simulink model "compensacion_digital"  (R2014b)
settings: Solver=ode45  StartTime=0.0  StopTime=4  RelTol=1e-3
settings Model: Creator=Javi  LastModifiedBy=Javi

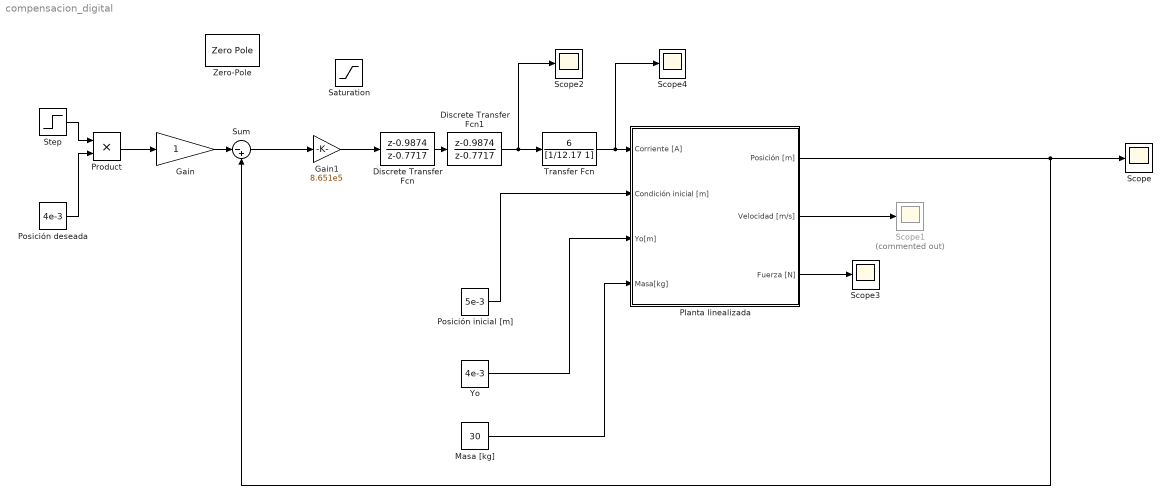
== system compensacion_digital ==
  Discrete Transfer Fcn : DiscreteTransferFcn  Numerator=[1 -0.9874]  Denominator=[1 -0.7717]  SampleTime=1/3.5e3
  Discrete Transfer Fcn1 : DiscreteTransferFcn  Numerator=[1 -0.9874]  Denominator=[1 -0.7717]
  Gain : Gain
  Gain1 : Gain  Gain=8.651e5
  "Masa [kg] " : Constant  Value=30
  Planta linealizada : Subsystem
  Posición deseada : Constant  Value=4e-3
  "Posición inicial [m] " : Constant  Value=5e-3
  Product : Product
  Saturation : Saturate  UpperLimit=5  LowerLimit=-inf
  Scope{,2..4} (4 alike) : Scope
      Scope settings: TimeRange=4  YMin=0  YMax=0.014
      Scope2 settings: TimeRange=0.005185185185185187  YMin=-3500000  YMax=500000  SaveName=ScopeData2
      Scope3 settings: TimeRange=4  YMin=-400000  YMax=600000  SaveName=ScopeData3
      Scope4 settings: TimeRange=0.005185185185185187  YMin=-3500000  YMax=500000  SaveName=ScopeData4
  Scope1 : Scope  Commented=on
  Step : Step  Time=0.01  SampleTime=0
  Sum : Sum  Inputs=|-+
  Transfer Fcn : TransferFcn  Numerator=[6]  Denominator=[1/12.17 1]
  "Yo " : Constant  Value=4e-3
  Zero-Pole : ZeroPole  Zeros=[-221.7 -221.7]  Poles=[-4511 -4511]  Gain=8.28e5
  wires:
  "Posición inicial [m] "/1 -> Planta linealizada/2("Condición inicial [m] ")
  "Yo "/1 -> Planta linealizada/3(Yo[m])
  "Masa [kg] "/1 -> Planta linealizada/4("Masa[kg] ")
  Planta linealizada/2(Velocidad [m/s]) -> Scope1/1
  Gain/1 -> Sum/1
  Planta linealizada/1(Posición [m]) -> Sum/2, Scope/1
  Transfer Fcn/1 -> Scope4/1, Planta linealizada/1(Corriente [A])
  Planta linealizada/3(Fuerza [N]) -> Scope3/1
  Discrete Transfer Fcn1/1 -> Scope2/1, Transfer Fcn/1
  Step/1 -> Product/1
  Posición deseada/1 -> Product/2
  Product/1 -> Gain/1
  Gain1/1 -> Discrete Transfer Fcn/1
  Sum/1 -> Gain1/1
  Discrete Transfer Fcn/1 -> Discrete Transfer Fcn1/1

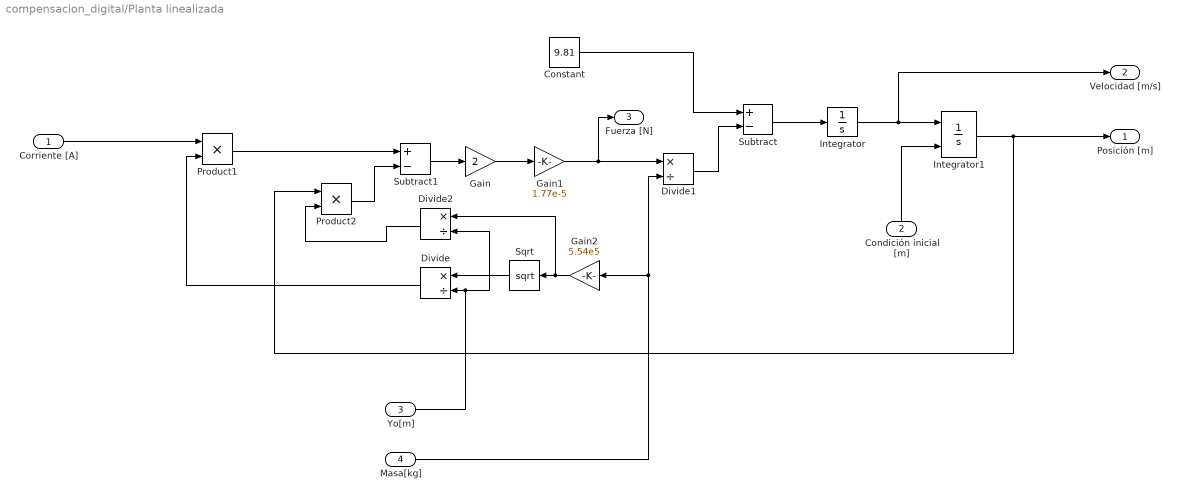
== system compensacion_digital/Planta linealizada ==
  Corriente [A] : Inport
  "Condición inicial [m] " : Inport  Port=2
  Yo[m] : Inport  Port=3
  "Masa[kg] " : Inport  Port=4
  Constant : Constant  Value=9.81
  Divide : Product  Inputs=*/
  Divide1 : Product  Inputs=*/
  Divide2 : Product  Inputs=*/
  Gain : Gain  Gain=2
  Gain1 : Gain  Gain=1.77e-5
  Gain2 : Gain  Gain=5.54e5
  Integrator : Integrator
  Integrator1 : Integrator  InitialConditionSource=external  LimitOutput=on  LowerSaturationLimit=0
  Product1 : Product
  Product2 : Product
  Sqrt : Sqrt  SaturateOnIntegerOverflow=on
  Subtract : Sum  Inputs=+-
  Subtract1 : Sum  Inputs=+-
  Posición [m] : Outport
  Velocidad [m/s] : Outport  Port=2
  Fuerza [N] : Outport  Port=3
  wires:
  Divide1/1 -> Subtract/2
  Gain2/1 -> Divide2/1, Sqrt/1
  Product1/1 -> Subtract1/1
  Corriente [A]/1 -> Product1/1
  Sqrt/1 -> Divide/1
  Yo[m]/1 -> Divide2/2, Divide/2
  Product2/1 -> Subtract1/2
  Divide/1 -> Product1/2
  Divide2/1 -> Product2/2
  "Masa[kg] "/1 -> Gain2/1, Divide1/2
  "Condición inicial [m] "/1 -> Integrator1/2
  Integrator/1 -> Velocidad [m/s]/1, Integrator1/1
  Integrator1/1 -> Posición [m]/1, Product2/1
  Subtract/1 -> Integrator/1
  Subtract1/1 -> Gain/1
  Gain/1 -> Gain1/1
  Gain1/1 -> Fuerza [N]/1, Divide1/1
  Constant/1 -> Subtract/1
